simulink model "Lab06"  (R2023b)
settings: Solver=VariableStepAuto  StartTime=0.0  StopTime=10  RelTol=1e-3
libraries: spsDCVoltageSourceLib x2, spsDCMachineLib x1, sps_lib x1
settings Model: Creator=sarth  LastModifiedBy=sarth

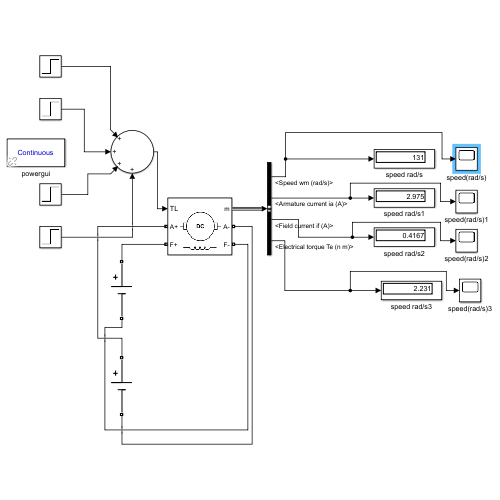
[thumbnail: Simulink's stored preview of the top-level diagram]
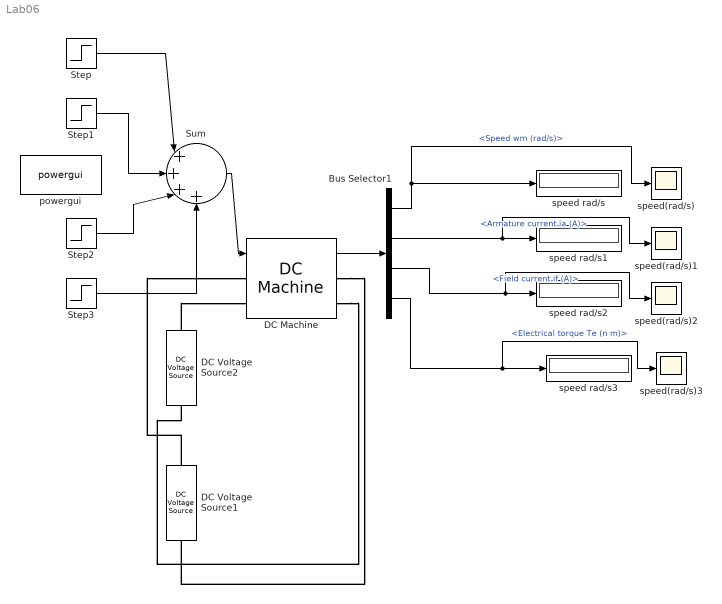
== system Lab06 ==
  Bus Selector1 : BusSelector  OutputSignals=Speed wm (rad/s),Armature current ia (A),Field current if (A),Electrical torque Te (n m)
  DC Machine : spsDCMachineLib/DC Machine  PresetModel=No  MechanicalLoad=Torque TL  FieldType=Wound  ShowDetailedParameters=on  MeasurementBus=off  RLa="[ 0.6  0.012]"  RLf="[ 240  120]"  Laf=1.8  MachineConstant=Torque constant (N.m/A)  Ke=1.8  Kt=1.8  J=1  Bm=0  Tf=0  w0=1  Ifinit=0.416666666666667  TsPowergui=0  TsBlock=-1
  DC Voltage Source1 : spsDCVoltageSourceLib/DC Voltage Source  Amplitude=100  Measurements=None
  DC Voltage Source2 : spsDCVoltageSourceLib/DC Voltage Source  Amplitude=100  Measurements=None
  Step : Step  Time=2.5  After=0.25  SampleTime=0
  Step1 : Step  Time=5  Before=0.25  After=0.50  SampleTime=0
  Step2 : Step  Time=7.5  Before=0.5  After=0.75  SampleTime=0
  Step3 : Step  Time=10  Before=0.75  SampleTime=0
  Sum : Sum  Inputs=|++++
  powergui : sps_lib/powergui  Priority=1  SimulationMode=Continuous  SampleTime=50e-6  frequency=60  Iterations=50  frequencyindice=0  Pbase=100e6  ErrMax=1e-4  UnitsV=kV  UnitsW=MW  buscounter=0  FunctionMessages=off  echomessages=off  EnableUseOfTLC=off  CurrentSourceSwitches=off  DisableSnubberDevices=off  DisableRonSwitches=off  DisableVfSwitches=off  DisplayEquations=off  AutomaticDiscreteSolvers=off  SolverType=Tustin/Backward Euler (TBE)  Interpol=off  ExternalGateDelay=off  methode=off  Ts=100  x0status=blocks  SPID=on  SwTol=0  HookPort=off  NonlinearTolerance=1e-4  nMaxIteration=100  ContinueOnMaxIteration=off  RestoreLinks=warning  ResistiveCurrentMeasurement=off  Frange=[0:2:500]  Ylog=off  Xlog=on  ShowGrid=off  save=off  variable=ZData  structure=0  ZoomFFT=off  StartTime=0.0  cycles=1  DisplayStyle=1  fundamental=60  FreqAxis=off  MaxFrequency=1000  frequencyindicesteady=1  RmsSteady=1  display=off
  speed rad/s{,1..3} (4 alike) : Display
  speed(rad/s){,1..3} (4 alike) : Scope
  wires:
  Step3/1 -> Sum/4
  Step1/1 -> Sum/2
  Step2/1 -> Sum/3
  DC Machine/1 -> Bus Selector1/1
  Step/1 -> Sum/1
  Sum/1 -> DC Machine/1
  Bus Selector1/1 -> speed rad/s/1, speed(rad/s)/1  "<Speed wm (rad/s)>"
  Bus Selector1/2 -> speed(rad/s)1/1, speed rad/s1/1  "<Armature current ia (A)>"
  Bus Selector1/3 -> speed(rad/s)2/1, speed rad/s2/1  "<Field current if (A)>"
  Bus Selector1/4 -> speed(rad/s)3/1, speed rad/s3/1  "<Electrical torque Te (n m)>"
  connections:
  DC Machine/RConn2 -- DC Voltage Source2/LConn1
  DC Voltage Source2/RConn1 -- DC Machine/LConn2
  DC Voltage Source1/RConn1 -- DC Machine/LConn1
  DC Machine/RConn1 -- DC Voltage Source1/LConn1
